simulink model "Arduino_MPU6050"  (R2021b)
settings: Solver=FixedStepDiscrete  StartTime=0.0  StopTime=inf  RelTol=1e-3  EnableMultiTasking=on
PostLoadFcn:
  | Simulink.importExternalCTypes('wire.h', 'EnumClass', 'dynamic');
undefined symbols (not defined in the file): DiscIntNeverNeededParam
libraries: arduinolib x10, simulink x1
settings Model: SimulationMode=external  ExtModeBatchMode=on  ExtModeTrigDuration=2  Creator=khoi  LastModifiedBy=khoi
settings OptimizationCC: UseDivisionForNetSlopeComputation=on  GainParamInheritBuiltInType=on  UseFloatMulNetSlope=on  DefaultUnderspecifiedDataType=single  PassReuseOutputArgsAs=Individual arguments  ZeroExternalMemoryAtStartup=off  ZeroInternalMemoryAtStartup=off  NoFixptDivByZeroProtection=on  EfficientFloat2IntCast=on  LifeSpan=1  MaxStackSize=64  OptimizeBlockOrder=speed  DifferentSizesBufferReuse=on  EfficientTunableParamExpr=on
settings DebuggingCC: ParameterTunabilityLossMsg=error
settings HardwareCC: ProdBitPerInt=16  ProdBitPerPointer=16  ProdBitPerSizeT=16  ProdBitPerPtrDiffT=16  ProdLargestAtomicFloat=None  ProdWordSize=8  ProdHWDeviceType=Atmel->AVR
settings ModelReferenceCC: EnableParallelModelReferenceBuilds=on
settings SFSimCC: MATLABDynamicMemAlloc=off  SimTargetLang=C++
settings RTWCC: Description=Embedded Coder  SystemTargetFile=ert.tlc  HardwareBoard=Arduino Mega 2560  TemplateMakefile=ert_default_tmf  Toolchain=Arduino AVR  BuildConfiguration=Faster Runs
settings CodeAppCC: ForceParamTrailComments=on  IgnoreCustomStorageClasses=off  OperatorAnnotations=on  SimulinkDataObjDesc=on  SFDataObjDesc=on  CustomSymbolStrGlobalVar=rt$N$M  CustomSymbolStrType=$N$M  CustomSymbolStrFcn=$N$M$F  CustomSymbolStrMacro=$N$M  InsertBlockDesc=on
settings ERTTargetCC: TargetLangStandard=C99 (ISO)  IncludeMdlTerminateFcn=off  CombineSignalStateStructs=on  SupportNonFinite=off  SupportComplex=off  SupportVariableSizeSignals=on  ExtMode=on  ExtModeTransport=3  ExtModeStaticAlloc=on  ExtModeStaticAllocSize=2048  ExtModeMexFile=ext_xcp  ExtModeMexArgs=0 3 921600  ExtModeIntrfLevel=Level2 - Open  ERTFilePackagingFormat=CompactWithDataFile

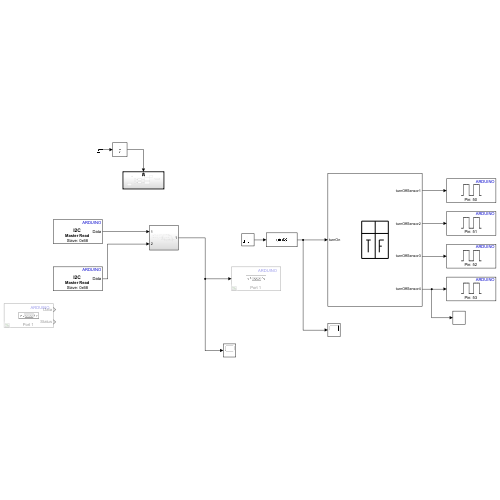
[thumbnail: Simulink's stored preview of the top-level diagram]
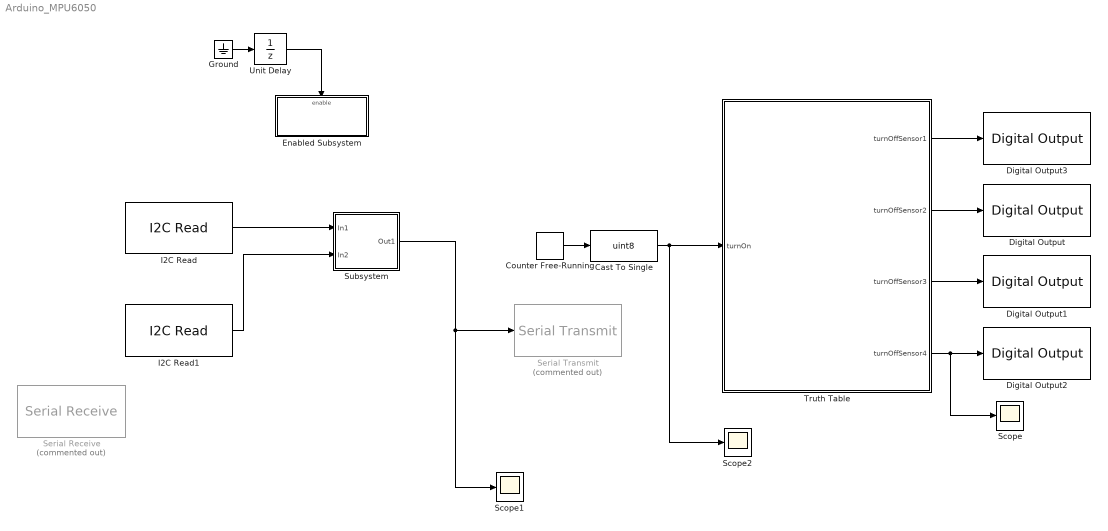
== system Arduino_MPU6050 ==
  Cast To Single : DataTypeConversion  OutDataTypeStr=uint8
  Counter Free-Running : simulink/Sources/Counter Free-Running  NumBits=2  tsamp=0.02
  Digital Output : arduinolib/Digital Output  pinNumber=51  Direction=output  blockPlatform=arduino
  Digital Output1 : arduinolib/Digital Output  pinNumber=52  Direction=output  blockPlatform=arduino
  Digital Output2 : arduinolib/Digital Output  pinNumber=53  Direction=output  blockPlatform=arduino
  Digital Output3 : arduinolib/Digital Output  pinNumber=50  Direction=output  blockPlatform=arduino
  Enabled Subsystem : Subsystem  TreatAsAtomicUnit=on
  Ground : Ground
  I2C Read : arduinolib/I2C Read  I2CModule=0  Mode=Master  SlaveAddress=uint8(hex2dec('68'))  SlaveByteOrder=BigEndian  Direction=Receiver  RegisterAddressMode=on  RegisterAddress=uint8(hex2dec('3B'))  SlaveDataType=int16  DataLength=3  NoAck=off  RepeatedStart=off  OutputStatus=off  blockPlatform=ARDUINO  SampleTime=0.02
      settings: SourceProductBaseCode=ARDUINO
  I2C Read1 : arduinolib/I2C Read  I2CModule=0  Mode=Master  SlaveAddress=uint8(hex2dec('68'))  SlaveByteOrder=BigEndian  Direction=Receiver  RegisterAddressMode=on  RegisterAddress=uint8(hex2dec('43'))  SlaveDataType=int16  DataLength=3  NoAck=off  RepeatedStart=off  OutputStatus=off  blockPlatform=ARDUINO  SampleTime=0.02
      settings: SourceProductBaseCode=ARDUINO
  Scope : Scope
  Scope1 : Scope
  Scope2 : Scope
  Serial Receive : arduinolib/Serial Receive  Commented=on  isARMArch=off  portNumber=1  DataType=single  Datalength=3  SampleTime=0.02  showOutStatus=on  blockPlatform=arduino
      settings: SourceProductBaseCode=ARDUINO
  Serial Transmit : arduinolib/Serial Transmit  Commented=on  portNumber=1  sendmode=print  label=;  sendformat=Decimal  floatprecision=3  blockPlatform=arduino
  Subsystem : Subsystem
  Truth Table : Truth Table  TreatAsAtomicUnit=on
  Unit Delay : UnitDelay  InitialCondition=1  SampleTime=-1  HasFrameUpgradeWarning=on
  wires:
  Ground/1 -> Unit Delay/1
  Unit Delay/1 -> Enabled Subsystem/Enable
  I2C Read/1 -> Subsystem/1(In1)
  I2C Read1/1 -> Subsystem/2(In2)
  Cast To Single/1 -> Scope2/1, Truth Table/1(turnOn)
  Counter Free-Running/1 -> Cast To Single/1
  Subsystem/1(Out1) -> Scope1/1, Serial Transmit/1
  Truth Table/1(turnOffSensor1) -> Digital Output3/1
  Truth Table/2(turnOffSensor2) -> Digital Output/1
  Truth Table/3(turnOffSensor3) -> Digital Output1/1
  Truth Table/4(turnOffSensor4) -> Scope/1, Digital Output2/1

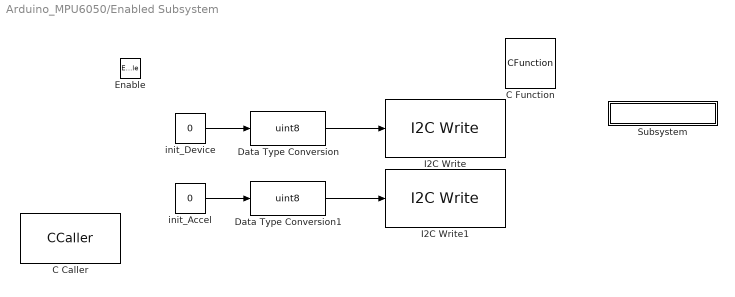
== system Arduino_MPU6050/Enabled Subsystem ==
  Enable : EnablePort
  C Caller : CCaller  FunctionName=setup
  C Function : CFunction
  Data Type Conversion : DataTypeConversion  OutDataTypeStr=uint8  RndMeth=Simplest
  Data Type Conversion1 : DataTypeConversion  OutDataTypeStr=uint8  RndMeth=Simplest
  I2C Write : arduinolib/I2C Write  I2CModule=0  Mode=Master  SlaveAddress=uint8(hex2dec('68'))  SlaveByteOrder=BigEndian  Direction=Transmitter  RegisterAddressMode=on  RegisterAddress=uint8(hex2dec('6B'))  SlaveDataType=uint8  DataLength=1  NoAck=off  RepeatedStart=off  OutputStatus=off  blockPlatform=ARDUINO
      settings: SourceProductBaseCode=ARDUINO
  I2C Write1 : arduinolib/I2C Write  I2CModule=0  Mode=Master  SlaveAddress=uint8(hex2dec('68'))  SlaveByteOrder=BigEndian  Direction=Transmitter  RegisterAddressMode=on  RegisterAddress=uint8(hex2dec('1C'))  SlaveDataType=uint8  DataLength=1  NoAck=off  RepeatedStart=off  OutputStatus=off  blockPlatform=ARDUINO
      settings: SourceProductBaseCode=ARDUINO
  Subsystem : Subsystem  mask{filename=wire.h}
      mask Display: disp('wire.h')
  init_Accel : Constant  Value=0
  init_Device : Constant  Value=0
  wires:
  init_Device/1 -> Data Type Conversion/1
  init_Accel/1 -> Data Type Conversion1/1
  Data Type Conversion/1 -> I2C Write/1
  Data Type Conversion1/1 -> I2C Write1/1

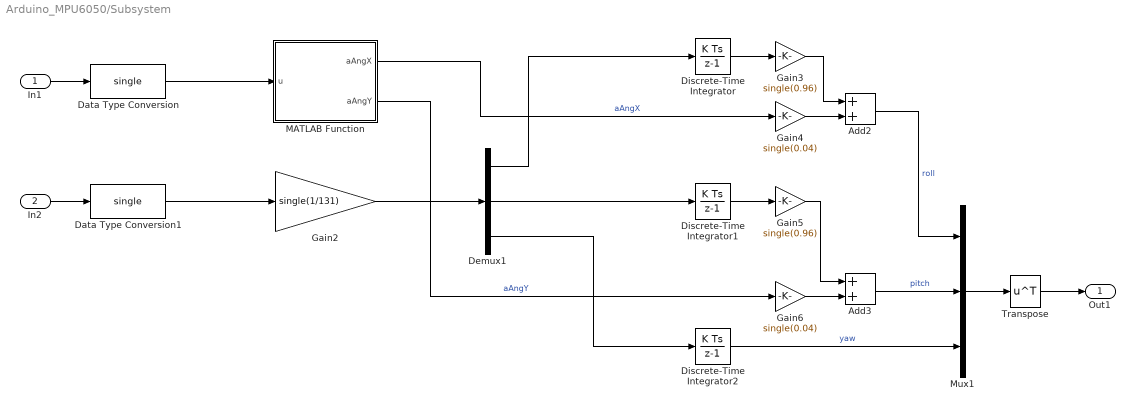
== system Arduino_MPU6050/Subsystem ==
  In1 : Inport
  In2 : Inport  Port=2
  Add2 : Sum
  Add3 : Sum
  Data Type Conversion : DataTypeConversion  OutDataTypeStr=single
  Data Type Conversion1 : DataTypeConversion  OutDataTypeStr=single
  Demux1 : Demux  Outputs=3
  Discrete-Time Integrator : DiscreteIntegrator  SampleTime=-1  ICPrevOutput=DiscIntNeverNeededParam  ICPrevScaledInput=DiscIntNeverNeededParam
  Discrete-Time Integrator1 : DiscreteIntegrator  SampleTime=-1  ICPrevOutput=DiscIntNeverNeededParam  ICPrevScaledInput=DiscIntNeverNeededParam
  Discrete-Time Integrator2 : DiscreteIntegrator  SampleTime=-1  ICPrevOutput=DiscIntNeverNeededParam  ICPrevScaledInput=DiscIntNeverNeededParam
  Gain2 : Gain  Gain=single(1/131)
  Gain3 : Gain  Gain=single(0.96)
  Gain4 : Gain  Gain=single(0.04)
  Gain5 : Gain  Gain=single(0.96)  ParamDataTypeStr=single
  Gain6 : Gain  Gain=single(0.04)  ParamDataTypeStr=single
  MATLAB Function : MATLAB Function  TreatAsAtomicUnit=on
  Mux1 : Mux  Inputs=3
  Transpose : Math  Operator=transpose  SaturateOnIntegerOverflow=on
  Out1 : Outport
  wires:
  MATLAB Function/2(aAngY) -> Gain6/1  "aAngY"
  Mux1/1 -> Transpose/1
  Add3/1 -> Mux1/2  "pitch"
  Demux1/1 -> Discrete-Time Integrator/1
  Gain3/1 -> Add2/1
  Gain4/1 -> Add2/2
  Add2/1 -> Mux1/1  "roll"
  Discrete-Time Integrator2/1 -> Mux1/3  "yaw"
  Discrete-Time Integrator/1 -> Gain3/1
  Discrete-Time Integrator1/1 -> Gain5/1
  Gain6/1 -> Add3/2
  Gain5/1 -> Add3/1
  Demux1/3 -> Discrete-Time Integrator2/1
  Demux1/2 -> Discrete-Time Integrator1/1
  Gain2/1 -> Demux1/1
  Data Type Conversion1/1 -> Gain2/1
  In2/1 -> Data Type Conversion1/1
  In1/1 -> Data Type Conversion/1
  Data Type Conversion/1 -> MATLAB Function/1(u)
  MATLAB Function/1(aAngX) -> Gain4/1  "aAngX"
  Transpose/1 -> Out1/1

== system Arduino_MPU6050/Enabled Subsystem/Subsystem ==

== matlab function Arduino_MPU6050/Truth Table ==
  data: turnOn input uint8; turnOffSensor1 output boolean; turnOffSensor2 output boolean; turnOffSensor3 output boolean; turnOffSensor4 output boolean
function [turnOffSensor1,turnOffSensor2, turnOffSensor3, turnOffSensor4] = fcn(turnOn)

aVarTruthTableCondition_1 = false;
aVarTruthTableCondition_2 = false;
aVarTruthTableCondition_3 = false;
aVarTruthTableCondition_4 = false;


% Accelerometer 1

aVarTruthTableCondition_1 = logical(turnOn==uint8(0));

% Accelerometer 2

aVarTruthTableCondition_2 = logical(turnOn==uint8(1));

% Accelerometer 3

aVarTruthTableCondition_3 = logical(turnOn==uint8(2));

% Accelerometer 4

aVarTruthTableCondition_4 = logical(turnOn==uint8(3));

if (aVarTruthTableCondition_1 && ~aVarTruthTableCondition_2 && ~aVarTruthTableCondition_3 && ~aVarTruthTableCondition_4)
    Sensor1On();
elseif (~aVarTruthTableCondition_1 && aVarTruthTableCondition_2 && ~aVarTruthTableCondition_3 && ~aVarTruthTableCondition_4)
    Sensor2On();
elseif (~aVarTruthTableCondition_1 && ~aVarTruthTableCondition_2 && aVarTruthTableCondition_3 && ~aVarTruthTableCondition_4)
    Sensor3On();
elseif (~aVarTruthTableCondition_1 && ~aVarTruthTableCondition_2 && ~aVarTruthTableCondition_3 && aVarTruthTableCondition_4)
    Sensor4On();
else % Default
    SensorError();
end

function Sensor1On()

% SNSR1

turnOffSensor1 = false;
turnOffSensor2 = true;
turnOffSensor3 = true;
turnOffSensor4 = true;

function Sensor2On()

% SNSR2

turnOffSensor1 = true;
turnOffSensor2 = false;
turnOffSensor3 = true;
turnOffSensor4 = true;

function Sensor3On()

% SNSR3

turnOffSensor1 = true;
turnOffSensor2 = true;
turnOffSensor3 = false;
turnOffSensor4 = true;

function Sensor4On()

% SNSR4

turnOffSensor1 = true;
turnOffSensor2 = true;
turnOffSensor3 = true;
turnOffSensor4 = false;

function SensorError()

% Error

turnOffSensor1 = true;
turnOffSensor2 = true;
turnOffSensor3 = true;
turnOffSensor4 = true;

== matlab function Arduino_MPU6050/Subsystem/MATLAB Function ==
  data: u input; aAngX output; aAngY output
function [aAngX,aAngY] = fcn(u)
aX=u(1)/16384; aY=u(2)/16384; aZ=u(3)/16384;
aAngX = atan(aY / sqrt(aX^2+aZ^2))*180/pi - 0.58;
aAngY = atan(-aX/ sqrt(aY^2+aZ^2))*180/pi + 1.58;
